simulink model "modelo_electrico_y_mecanico"  (R2023b)
settings: Solver=VariableStepAuto  StartTime=0.0  StopTime=10.0  RelTol=1e-3
PreLoadFcn:
  | Jcm=0.0208;
values from neighbouring files (symbols this model uses):
  b_l = 0.1    [polos_y_ceros.m]    (also in var1.m = 0.2)
  g = 9.80665    [polos_y_ceros.m]    (also in var1.m = 9.8)
  J_cm = 0.0208    [polos_y_ceros.m]    (also in var1.m)
  k_l = m * L_cm + m_l * L_l    (= 0.25)    [polos_y_ceros.m]    (also in var1.m = 1)
  L_d = 6.6 * 10^(-3)    (= 0.0066)    [polos_y_ceros.m]    (also in var1.m = 6.6)
  L_q = 5.8 * 10^(-3)    (= 0.0058)    [polos_y_ceros.m]    (also in var1.m = 5.8)
  lambda_m = 0.016    [polos_y_ceros.m]    (also in var1.m)
  P_p = 3    [polos_y_ceros.m]    (also in var1.m)
settings Model: Creator=tomas  LastModifiedBy=gonza

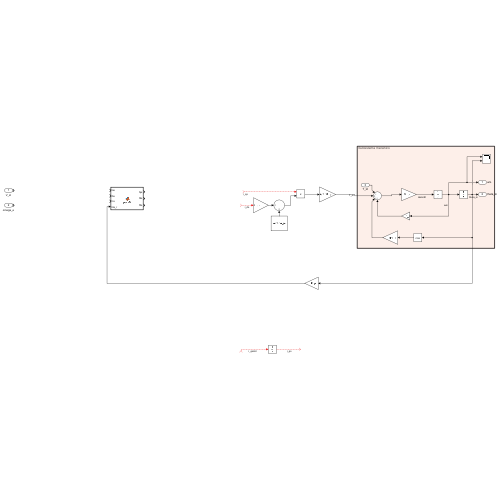
[thumbnail: Simulink's stored preview of the top-level diagram]
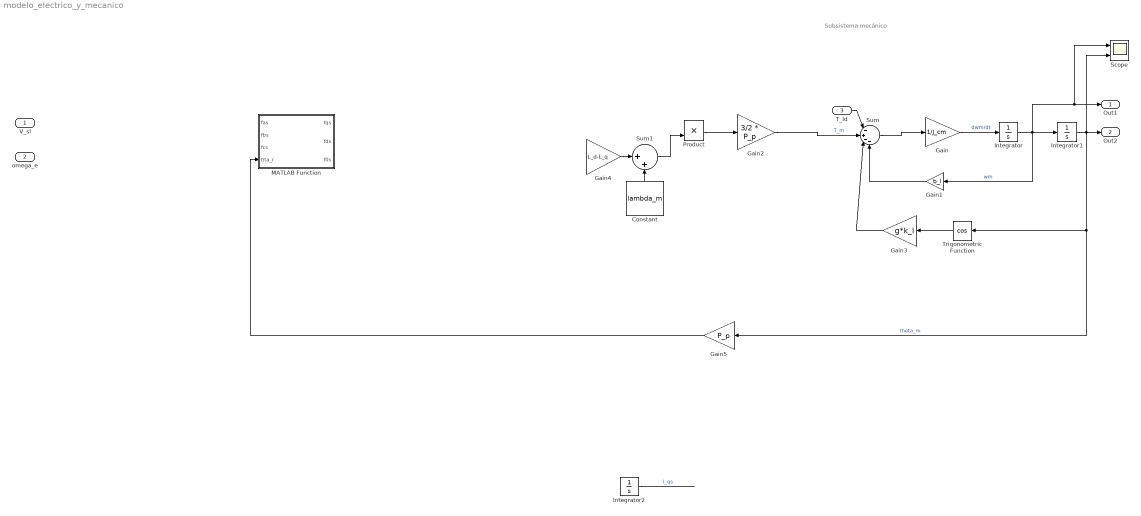
== system modelo_electrico_y_mecanico ==
  note: Subsistema mecánico
  V_sl : Inport
  omega_e : Inport  Port=2
  T_ld : Inport  Port=3
  Constant : Constant  Value=lambda_m
  Gain : Gain  Gain=1/J_cm
  Gain1 : Gain  Gain=b_l
  Gain2 : Gain  Gain=3/2 * P_p
  Gain3 : Gain  Gain=g*k_l
  Gain4 : Gain  Gain=L_d-L_q
  Gain5 : Gain  Gain=P_p
  Integrator : Integrator
  Integrator1 : Integrator
  Integrator2 : Integrator
  MATLAB Function : MATLAB Function  TreatAsAtomicUnit=on
  Product : Product
  Scope : Scope  NumInputPorts=2
  Sum : Sum  Inputs=|-+--
  Sum1 : Sum  Inputs=|++
  Trigonometric Function : Trigonometry  Operator=cos
  Out1 : Outport  SignalName=wm
  Out2 : Outport  Port=2  SignalName=theta_m
  wires:
  Sum/1 -> Gain/1
  Gain/1 -> Integrator/1  "dwm/dt"
  Integrator/1 -> Gain1/1, Integrator1/1, Out1/1, Scope/1  "wm"
  Integrator1/1 -> Gain5/1, Trigonometric Function/1, Out2/1, Scope/2  "theta_m"
  T_ld/1 -> Sum/1
  Trigonometric Function/1 -> Gain3/1
  Gain1/1 -> Sum/4
  Gain3/1 -> Sum/3
  Gain2/1 -> Sum/2  "T_m"
  ? -> Product/1  "i_qs"
  ? -> Gain4/1  "i_ds"
  Product/1 -> Gain2/1
  Sum1/1 -> Product/2
  Gain4/1 -> Sum1/1
  Constant/1 -> Sum1/2
  Gain5/1 -> MATLAB Function/4(tita_r)
  Integrator2/1 -> ?  "i_qs"
  ? -> Integrator2/1  "i_qsdot"

== matlab function modelo_electrico_y_mecanico/MATLAB Function ==
  data: fas input; fqs output; fbs input; fcs input; tita_r input; fds output; f0s output
function [fqs, fds, f0s]= parkD(fas,fbs,fcs,tita_r)
answer = 2/3 * [cos(tita_r),cos(tita_r-2*pi/3),cos(tita_r-2*pi/3);sin(tita_r),sin(tita_r-2*pi/3),sin(tita_r+2*pi/3);0.5,0.5,0.5] * [fas;fbs;fcs]; 
fqs = answer(1);
fds = answer(2);
f0s = answer(3);
